simulink model "untitled"  (R2014b)
settings: Solver=ode45  StartTime=0.0  StopTime=10.0  RelTol=1e-3
settings Model: Creator=user  LastModifiedBy=user

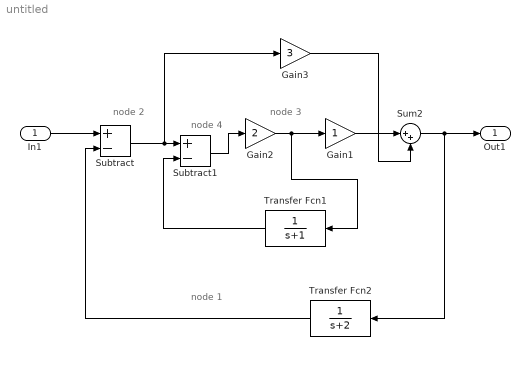
== system untitled ==
  note: node 2
  note: node 1
  note: node 4
  note: node 3
  In1 : Inport
  Gain1 : Gain
  Gain2 : Gain  Gain=2
  Gain3 : Gain  Gain=3
  Subtract : Sum  Inputs=+-
  Subtract1 : Sum  Inputs=+-
  Sum2 : Sum  Inputs=|++
  Transfer Fcn1 : TransferFcn  Denominator=[1 1]
  Transfer Fcn2 : TransferFcn  Denominator=[1 2]
  Out1 : Outport
  wires:
  In1/1 -> Subtract/1
  Sum2/1 -> Transfer Fcn2/1, Out1/1
  Transfer Fcn2/1 -> Subtract/2
  Subtract/1 -> Gain3/1, Subtract1/1
  Gain3/1 -> Sum2/2
  Gain1/1 -> Sum2/1
  Gain2/1 -> Transfer Fcn1/1, Gain1/1
  Transfer Fcn1/1 -> Subtract1/2
  Subtract1/1 -> Gain2/1
